simulink model "induction_machine"  (R2018b)
settings: Solver=VariableStepAuto  StartTime=0.0  StopTime=0.6  RelTol=1e-3
values from neighbouring files (symbols this model uses):
  load_tL = 3    [sim_induction_machine.m]
  P = 4    [sim_induction_machine.m]
  r_rp = dut.r_rp    [sim_induction_machine.m]
  r_s = dut.r_s    [sim_induction_machine.m]
  v_pk = v_rms*sqrt(2/3)    [sim_induction_machine.m]
  vs_toff = 3    [sim_induction_machine.m]
  w_b = 2*pi*f    (= 376.991118431)    [sim_induction_machine.m]
settings Model: Creator=carlo  LastModifiedBy=carlo

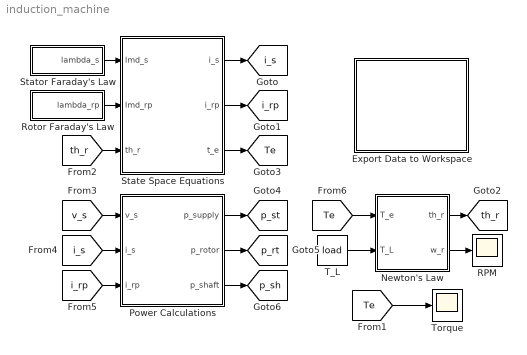
== system induction_machine ==
  Export Data to Workspace : Subsystem
  Newton's Law : Subsystem
  Power Calculations : MATLAB Function  TreatAsAtomicUnit=on
  RPM : Scope
  Rotor Faraday's Law : Subsystem
  State Space Equations : MATLAB Function  TreatAsAtomicUnit=on
  Stator Faraday's Law : Subsystem
  T_L : Constant  Value=load
  Torque : Scope
  tag scope: Te=global, i_rp=global, i_s=global, p_rt=global, p_sh=global, p_st=global, th_r=global
  wires:
  Newton's Law/1(th_r) -> [th_r]
  Newton's Law/2(w_r) -> RPM/1
  [th_r] -> State Space Equations/3(th_r)
  State Space Equations/1(i_s) -> [i_s]
  State Space Equations/2(i_rp) -> [i_rp]
  Rotor Faraday's Law/1(lambda_rp) -> State Space Equations/2(lmd_rp)
  Stator Faraday's Law/1(lambda_s) -> State Space Equations/1(lmd_s)
  [v_s] -> Power Calculations/1(v_s)
  [i_s] -> Power Calculations/2(i_s)
  [i_rp] -> Power Calculations/3(i_rp)
  Power Calculations/1(p_supply) -> [p_st]
  Power Calculations/2(p_rotor) -> [p_rt]
  Power Calculations/3(p_shaft) -> [p_sh]
  State Space Equations/3(t_e) -> [Te]
  [Te] -> Newton's Law/1(T_e)
  [Te] -> Torque/1
  T_L/1 -> Newton's Law/2(T_L)

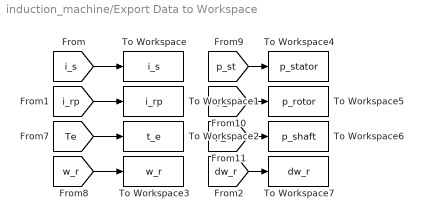
== system induction_machine/Export Data to Workspace ==
  To Workspace : ToWorkspace  VariableName=i_s  SaveFormat=Timeseries  SampleTime=-1
  To Workspace1 : ToWorkspace  VariableName=i_rp  SaveFormat=Timeseries  SampleTime=-1
  To Workspace2 : ToWorkspace  VariableName=t_e  SaveFormat=Timeseries  SampleTime=-1
  To Workspace3 : ToWorkspace  VariableName=w_r  SaveFormat=Timeseries  SampleTime=-1
  To Workspace4 : ToWorkspace  VariableName=p_stator  SaveFormat=Timeseries  SampleTime=-1
  To Workspace5 : ToWorkspace  VariableName=p_rotor  SaveFormat=Timeseries  SampleTime=-1
  To Workspace6 : ToWorkspace  VariableName=p_shaft  SaveFormat=Timeseries  SampleTime=-1
  To Workspace7 : ToWorkspace  VariableName=dw_r  SaveFormat=Timeseries  SampleTime=-1
  wires:
  [p_rt] -> To Workspace5/1
  [p_st] -> To Workspace4/1
  [Te] -> To Workspace2/1
  [i_s] -> To Workspace/1
  [w_r] -> To Workspace3/1
  [i_rp] -> To Workspace1/1
  [p_sh] -> To Workspace6/1
  [dw_r] -> To Workspace7/1

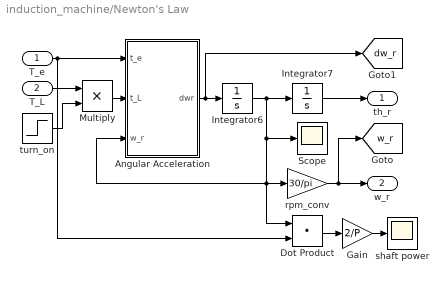
== system induction_machine/Newton's Law ==
  T_e : Inport
  T_L : Inport  Port=2
  Angular Acceleration : MATLAB Function  TreatAsAtomicUnit=on
  Dot Product : DotProduct  InputSameDT=on  OutDataTypeStr=Inherit: Inherit via internal rule
  Gain : Gain  Gain=2/P
  Integrator6 : Integrator
  Integrator7 : Integrator
  Multiply : Product
  Scope : Scope
  rpm_conv : Gain  Gain=30/pi
  shaft power : Scope
  turn_on : Step  Time=load_tL  SampleTime=0
  th_r : Outport
  w_r : Outport  Port=2
  tag scope: dw_r=global, w_r=global
  wires:
  Integrator6/1 -> Scope/1, Angular Acceleration/3(w_r), rpm_conv/1, Dot Product/1, Integrator7/1
  Integrator7/1 -> th_r/1
  rpm_conv/1 -> w_r/1, [w_r]
  T_e/1 -> Dot Product/2, Angular Acceleration/1(t_e)
  Angular Acceleration/1(dwr) -> [dw_r], Integrator6/1
  Multiply/1 -> Angular Acceleration/2(t_L)
  T_L/1 -> Multiply/1
  turn_on/1 -> Multiply/2
  Dot Product/1 -> Gain/1
  Gain/1 -> shaft power/1

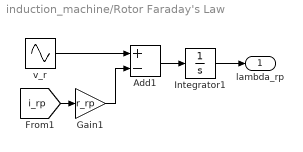
== system induction_machine/Rotor Faraday's Law ==
  Add1 : Sum  Inputs=+-
  Gain1 : Gain  Gain=r_rp
  Integrator1 : Integrator
  v_r : Sin  Amplitude=0  Frequency=w_b  Phase=[0;-1;1]*2*pi/3  SampleTime=0
  lambda_rp : Outport
  wires:
  [i_rp] -> Gain1/1
  Integrator1/1 -> lambda_rp/1
  Add1/1 -> Integrator1/1
  Gain1/1 -> Add1/2
  v_r/1 -> Add1/1

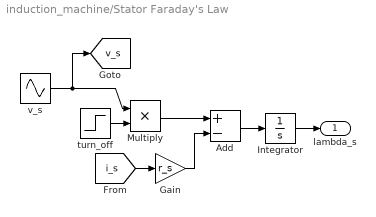
== system induction_machine/Stator Faraday's Law ==
  Add : Sum  Inputs=+-
  Gain : Gain  Gain=r_s
  Integrator : Integrator
  Multiply : Product
  turn_off : Step  Time=vs_toff  Before=1  After=0  SampleTime=0
  v_s : Sin  Amplitude=v_pk  Frequency=w_b  Phase=[0;-1;1]*2*pi/3  SampleTime=0
  lambda_s : Outport
  tag scope: v_s=global
  wires:
  Integrator/1 -> lambda_s/1
  Add/1 -> Integrator/1
  Gain/1 -> Add/2
  [i_s] -> Gain/1
  v_s/1 -> Multiply/1, [v_s]
  turn_off/1 -> Multiply/2
  Multiply/1 -> Add/1

== matlab function induction_machine/Power Calculations ==
  data: v_s input; i_s input; i_rp input; params parameter; p_supply output; p_rotor output; p_shaft output
function [p_supply,p_rotor,p_shaft] = pwr(v_s,i_s,i_rp,params)
%% Unpacking parameters
r_s = params(5);
r_rp = params(6);
%% Initial Power
p_supply = dot(v_s,i_s);            % Power in supplied
%% Stator Losses
p_sl = sum(r_s*i_s.^2);             % losses due to stator
%% Rotor Losses
p_rl = sum(r_rp*i_rp.^2);           % losses due to rotor
%% Calculations
p_shaft = p_supply - p_sl - p_rl;   % Power in shaft
p_rotor = p_supply - p_sl;          % Power in rotor

== matlab function induction_machine/State Space Equations ==
  data: lmd_s input; lmd_rp input; th_r input; i_s output; params parameter; i_rp output; t_e output
function [i_s,i_rp,t_e] = state_eqs(lmd_s, lmd_rp,th_r, params)
%% Unpacking parameters
L_ls = params(1);
L_ms = params(2);
L_lr_p = params(3);
P = params(4);
%% Inductance Matrices
off_diag = -0.5*L_ms;
% Stator
L_s = [
    L_ls+L_ms off_diag off_diag;
    off_diag L_ls+L_ms off_diag;
    off_diag off_diag L_ls+L_ms];
% Referred Rotor
L_rp = [
    L_lr_p+L_ms off_diag off_diag;
    off_diag L_lr_p+L_ms off_diag;
    off_diag off_diag L_lr_p+L_ms];
%% Mutual Inductance Matrix
o = 2*pi/3;
L_sr = L_ms*[
    cos(th_r) cos(th_r+o) cos(th_r-o);
    cos(th_r-o) cos(th_r) cos(th_r+o);
    cos(th_r+o) cos(th_r-o) cos(th_r)];
%% Inductance matrix
L = [L_s L_sr;
     L_sr' L_rp];
%% Vectorizing flux linkages
lam = [lmd_s;lmd_rp];
%% Calculating currents
i = L\lam;
%% Stator and Referred Rotor Currents
i_s = i(1:3);
i_rp = i(4:6);
%% Single current values
ias = i(1);ibs = i(2);ics = i(3);
iarp = i(4);ibrp = i(5);icrp = i(6);
%% Calculation of torque produced
t_e = -(P/2)*L_ms*(  ...
    (ias*(iarp-(1/2)*ibrp-(1/2)*icrp) ...
    +ibs*(ibrp-(1/2)*iarp-(1/2)*icrp) ...
    +ics*(icrp-(1/2)*ibrp-(1/2)*iarp))*sin(th_r) ...
    + (sqrt(3)/2)* ...
    (ias*(ibrp-icrp) ...
    +ibs*(icrp-iarp) ...
    +ics*(iarp-ibrp))*cos(th_r) ...
    );

== matlab function induction_machine/Newton's Law/Angular Acceleration ==
  data: t_e input; dwr output; t_L input; w_r input; params parameter
function dwr = dw_r(t_e,t_L,w_r,params)
%% Unpacking parameters
P = params(4);
J = params(7);
B = params(8);
%% Angular Acceleration
dwr = P*(t_e-t_L-B*w_r)/(2*J);
